simulink model "NRZ_DAC"  (Simulink 7.9)
settings: Solver=ode45  StartTime=0.0  StopTime=simu.trantime  RelTol=1e-3
undefined symbols (not defined in the file or in its folder): Fs
libraries: dspsigops x1
settings Model: Creator=amyles  LastModifiedBy=Arnaldi Isacco
settings SolverCC: ZeroCrossAlgorithm=Adaptive  AutoInsertRateTranBlk=on
settings DataIOCC: MaxDataPoints=50000  SaveOutput=off  SaveTime=off
settings OptimizationCC: InlineParams=on
settings DebuggingCC: UnderspecifiedInitializationDetection=Simplified  InvalidFcnCallConnMsg=none  StrictBusMsg=ErrorOnBusTreatedAsVector
settings ModelReferenceCC: ModelReferenceNumInstancesAllowed=Single
settings CodeAppCC: CustomSymbolStrType=$N$R$M_T
settings GRTTargetCC: CombineOutputUpdateFcns=off  GRTInterface=on

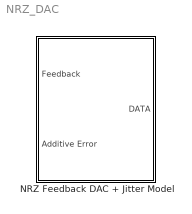
== system NRZ_DAC ==
  NRZ Feedback DAC + Jitter Model : Subsystem

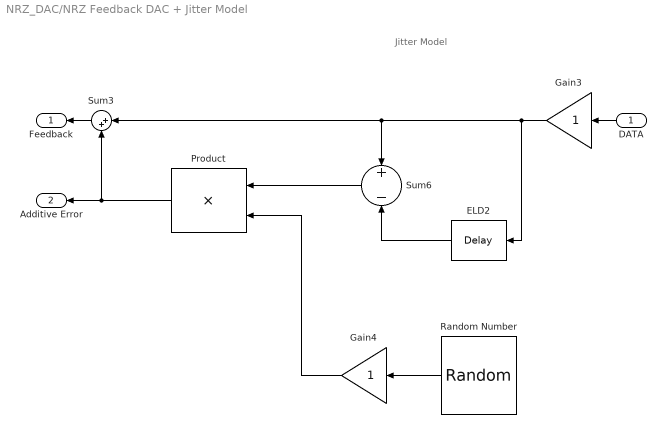
== system NRZ_DAC/NRZ Feedback DAC + Jitter Model ==
  note: Jitter Model
  DATA : Inport
  ELD2 : dspsigops/Delay  InputProcessing=Inherited (this choice will be removed - see release notes)  dly_unit=Samples  delay=1  ic_detail=off  dif_ic_for_ch=off  dif_ic_for_dly=off  ic=0  reset_popup=None
  Gain3 : Gain  SampleTime=1/Fs
  Gain4 : Gain  SampleTime=1/Fs
  Product : Product  SampleTime=1/Fs  RndMeth=Zero
  Random Number : RandomNumber  Mean=100e-12  Variance=50e-9  Seed=1  SampleTime=1/Fs
  Sum3 : Sum  Inputs=|++  SampleTime=1/Fs
  Sum6 : Sum  Inputs=+-  SampleTime=1/Fs
  Feedback : Outport
  Additive Error : Outport  Port=2
  wires:
  ELD2/1 -> Sum6/2
  Gain3/1 -> ELD2/1, Sum6/1, Sum3/1
  Sum6/1 -> Product/1
  Random Number/1 -> Gain4/1
  Gain4/1 -> Product/2
  Product/1 -> Sum3/2, Additive Error/1
  DATA/1 -> Gain3/1
  Sum3/1 -> Feedback/1
